simulink model "DiscretePulseGenerator_TestGen2"  (R2017b)
settings: Solver=FixedStepDiscrete  StartTime=0.0  StopTime=10.0  RelTol=1e-3
undefined symbols (not defined in the file): Block_TestLib, reset
settings Model: Creator=hbourbou  LastModifiedBy=hbourbou
settings DebuggingCC: ParameterOverflowMsg=none

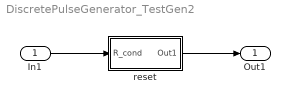
== system DiscretePulseGenerator_TestGen2 ==
  In1 : Inport
  reset : Subsystem  AncestorBlock=Block_TestLib/reset
  Out1 : Outport
  wires:
  In1/1 -> reset/1(R_cond)
  reset/1(Out1) -> Out1/1

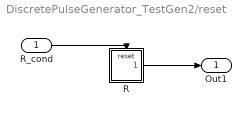
== system DiscretePulseGenerator_TestGen2/reset ==
  R_cond : Inport  OutDataTypeStr=boolean
  R : Subsystem  TreatAsAtomicUnit=on
  Out1 : Outport
  wires:
  R_cond/1 -> R/Reset
  R/1(Out1) -> Out1/1

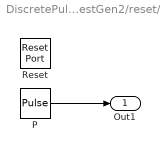
== system DiscretePulseGenerator_TestGen2/reset/R ==
  Reset : ResetPort  DisableCoverage=on
  P : DiscretePulseGenerator  PulseType=Time based  Amplitude=0.5  Period=5  PulseWidth=3  SampleTime=-1
  Out1 : Outport
  wires:
  P/1 -> Out1/1
